simulink model "FinalSimModel_Integrator"  (R2021b)
settings: Solver=VariableStepAuto  StartTime=0.0  StopTime=60  RelTol=1e-3
values from neighbouring files (symbols this model uses):
  Asfo = A - L*C    [ControllerDesignLQR.m]    (also in ControllerDesignLQR_WithIntegrator.m)
  Bsfo = [B-(L*D), L]    [ControllerDesignLQR.m]    (also in ControllerDesignLQR_WithIntegrator.m)
  Csfo = K    [ControllerDesignLQR.m]    (also in ControllerDesignLQR_WithIntegrator.m)
  Dsfo = zeros(1,2)    [ControllerDesignLQR.m]    (also in ControllerDesignLQR_WithIntegrator.m)
libraries: simulink x1
settings Model: Creator=randy  LastModifiedBy=randy

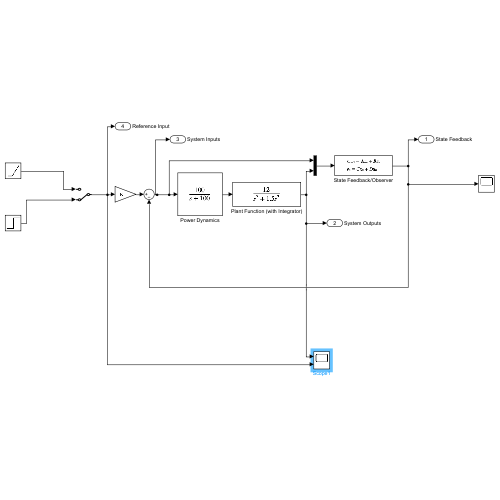
[thumbnail: Simulink's stored preview of the top-level diagram]
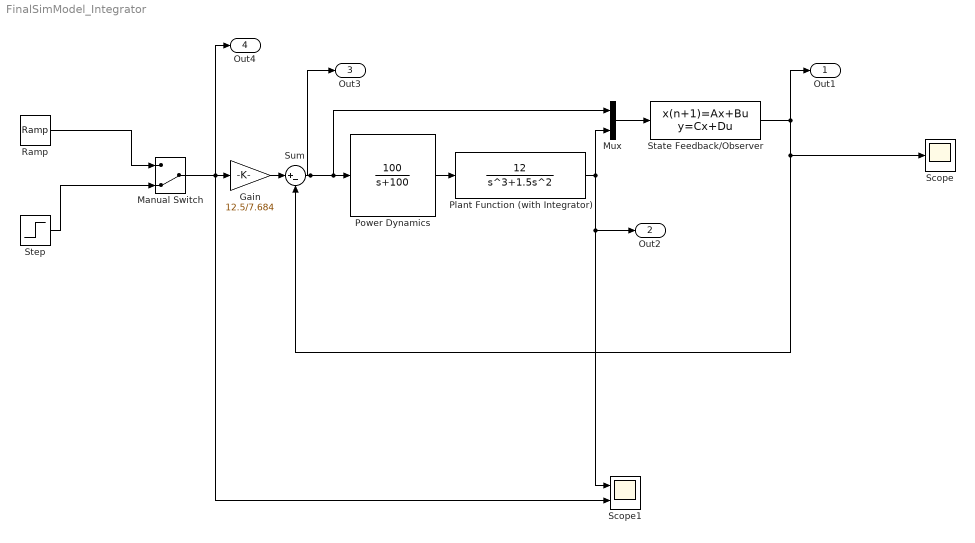
== system FinalSimModel_Integrator ==
  Gain : Gain  Gain=12.5/7.684
  Manual Switch : ManualSwitch  CurrentSetting=0
  Mux : Mux  Inputs=2
  Plant Function (with Integrator) : TransferFcn  Numerator=[12]  Denominator=[1 1.5 0 0]
  Power Dynamics : TransferFcn  Numerator=[100 ]  Denominator=[1 100 ]
  Ramp : simulink/Sources/Ramp  slope=0.78  start=0  InitialOutput=0
  Scope : Scope
  Scope1 : Scope  NumInputPorts=2
  State Feedback/Observer : DiscreteStateSpace  A=Asfo  B=Bsfo  C=Csfo  D=Dsfo  InitialCondition=2  SampleTime=0.05
  Step : Step  After=12.5  SampleTime=0
  Sum : Sum  Inputs=|+-
  Out1 : Outport  SignalName=State Feedback
  Out2 : Outport  Port=2  SignalName=System Outputs
  Out3 : Outport  Port=3  SignalName=System Inputs
  Out4 : Outport  Port=4  SignalName=Reference Input
  wires:
  State Feedback/Observer/1 -> Sum/2, Scope/1, Out1/1
  Mux/1 -> State Feedback/Observer/1
  Sum/1 -> Out3/1, Mux/1, Power Dynamics/1
  Manual Switch/1 -> Out4/1, Scope1/2, Gain/1
  Plant Function (with Integrator)/1 -> Scope1/1, Out2/1, Mux/2
  Gain/1 -> Sum/1
  Step/1 -> Manual Switch/2
  Power Dynamics/1 -> Plant Function (with Integrator)/1
  Ramp/1 -> Manual Switch/1
